simulink model "mod1"  (Simulink 8.9)
settings: Solver=ode45  StartTime=0.0  StopTime=simu.trantime  RelTol=1e-3  EnableMultiTasking=on
undefined symbols (not defined in the file): dc, Fs, mod, OSR, sinamp, sinfreq
libraries: dsparch4 x1, dspsrcs4 x1
settings Model: Creator=Isacco Arnaldi  LastModifiedBy=Arnaldi Isacco
settings SolverCC: AutoInsertRateTranBlk=on
settings DataIOCC: MaxDataPoints=50000  SaveOutput=off  SaveTime=off
settings OptimizationCC: DefaultParameterBehavior=Inlined  ExpressionDepthLimit=2147483647
settings DebuggingCC: SolverPrmCheckMsg=warning  StrictBusMsg=Warning

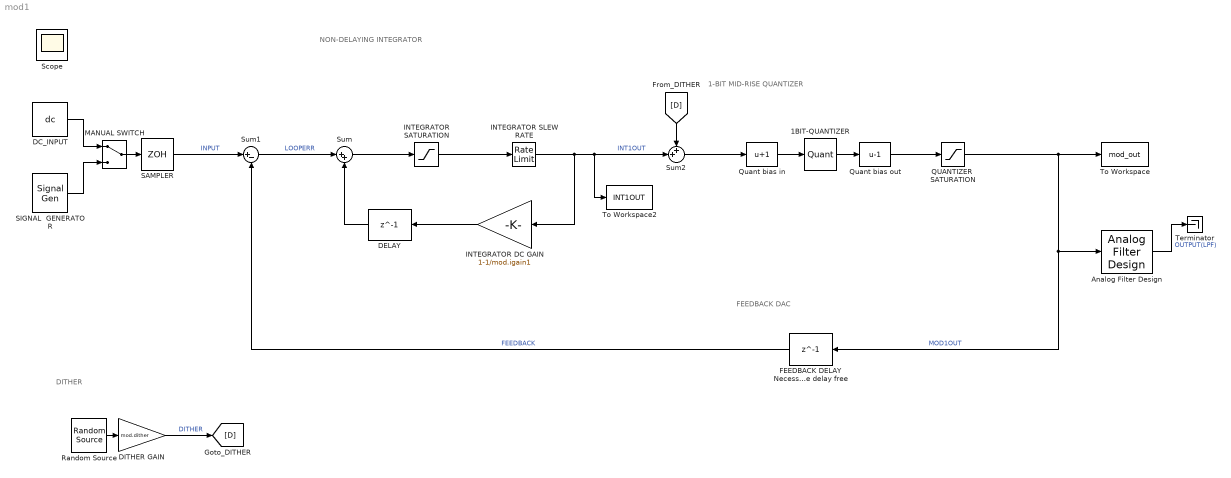
== system mod1 ==
  note: NON-DELAYING INTEGRATOR
  note: FEEDBACK DAC
  note: 1-BIT MID-RISE QUANTIZER
  note: DITHER
  1BIT-QUANTIZER : Quantizer  QuantizationInterval=2  LinearizeAsGain=off  SampleTime=1/Fs
      settings: AttributesFormatString=step = 2
  Analog Filter Design : dsparch4/Analog Filter Design  method=Butterworth  filttype=Lowpass  N=8  Wlo=pi*(Fs/OSR)  Whi=80  Rp=2  Rs=40
      settings: AttributesFormatString=Low-pass filter the loop output\nto illustrate intuitively how the\npulse density modulated +1/-1\noutput stream does indeed capture\nthe input signal
  DC_INPUT : Constant  Value=dc  OutDataTypeStr=double  SampleTime=1/Fs
  DELAY : Delay  DelayLength=1  InitialCondition=0  InputProcessing=Inherited
  DITHER GAIN : Gain  Gain=mod.dither  SampleTime=1/Fs
  FEEDBACK DELAY Necessary to avoid a delay-free loop as integrator and quantizer are delay free : Delay  DelayLength=1  InitialCondition=0  InputProcessing=Inherited
  INTEGRATOR SATURATION : Saturate  UpperLimit=mod.isat1  LowerLimit=-(mod.isat1)
      settings: AttributesFormatString=Real integrators will have\noutput swing limits (analog\nsignal headroom or digital\naccumulator min/max values)
  INTEGRATOR SLEW RATE : RateLimiter  RisingSlewLimit=mod.isr1  FallingSlewLimit=-(mod.isr1)  SampleTimeMode=inherited
      settings: AttributesFormatString=...and\nmay suffer from\npoor slew rate
  INTEGRATOR DC GAIN : Gain  Gain=1-1/mod.igain1
      settings: AttributesFormatString=Integrator leakage\n(model finite integrator dc/LF\ngain in analog modulators)
  MANUAL SWITCH : ManualSwitch
      settings: AttributesFormatString=Double click to\nselect the desired\ninput
  QUANTIZER  SATURATION : Saturate  UpperLimit=mod.qsatout1  LowerLimit=-(mod.qsatout1)
      settings: AttributesFormatString=Limit quantizer\noutput
  Quant bias in : Bias  Bias=1
      settings: AttributesFormatString=Need offset to give\nMID-RISE quantiser
  Quant bias out : Bias  Bias=-1
      settings: AttributesFormatString=Shift outputs to\n..., -2, 1, 1, ...
  Random Source : dspsrcs4/Random Source  SrcType=Uniform  NormMethod=Ziggurat  CltLength=12  MinVal=-1  MaxVal=1  MeanVal=0  VarVal=1  RepMode=Not repeatable  rawSeed=1  IsInherit=off  SampMode=Discrete  SampTime=1/Fs  SampFrame=1  DataType=Double  OutComplex=Real  OutputFrames=on
  SAMPLER : ZeroOrderHold  SampleTime=1/Fs
  SIGNAL  GENERATOR : SignalGenerator  Amplitude=sinamp  Frequency=sinfreq  VectorParams1D=off
  Sum : Sum  Inputs=|++
      settings: AttributesFormatString=Integrator\nsummer
  Sum1 : Sum  Inputs=|+-  SampleTime=1/Fs
      settings: AttributesFormatString=Modulator Input\nLoop Error (input - fbk)
  Sum2 : Sum  Inputs=++|
  Terminator : Terminator
  To Workspace : ToWorkspace  VariableName=mod_out  SampleTime=-1
      settings: AttributesFormatString=Export output to\nworkspace for\npost-processing
  To Workspace2 : ToWorkspace  VariableName=INT1OUT  SampleTime=-1
      settings: AttributesFormatString=Export output to\nworkspace for\npost-processing
  Scope : Scope
  wires:
  DELAY/1 -> Sum/2
  Sum/1 -> INTEGRATOR SATURATION/1
  Sum1/1 -> Sum/1  "LOOPERR"
  FEEDBACK DELAY Necessary to avoid a delay-free loop as integrator and quantizer are delay free/1 -> Sum1/2  "FEEDBACK"
  Random Source/1 -> DITHER GAIN/1
  INTEGRATOR DC GAIN/1 -> DELAY/1
  Quant bias out/1 -> QUANTIZER  SATURATION/1
  DITHER GAIN/1 -> [D]  "DITHER"
  Quant bias in/1 -> 1BIT-QUANTIZER/1
  1BIT-QUANTIZER/1 -> Quant bias out/1
  DC_INPUT/1 -> MANUAL SWITCH/1
  SIGNAL  GENERATOR/1 -> MANUAL SWITCH/2
  MANUAL SWITCH/1 -> SAMPLER/1
  Analog Filter Design/1 -> Terminator/1  "OUTPUT(LPF)"
  Sum2/1 -> Quant bias in/1
  [D] -> Sum2/1
  INTEGRATOR SLEW RATE/1 -> INTEGRATOR DC GAIN/1, To Workspace2/1, Sum2/2  "INT1OUT"
  INTEGRATOR SATURATION/1 -> INTEGRATOR SLEW RATE/1
  QUANTIZER  SATURATION/1 -> To Workspace/1, Analog Filter Design/1, FEEDBACK DELAY Necessary to avoid a delay-free loop as integrator and quantizer are delay free/1  "MOD1OUT"
  SAMPLER/1 -> Sum1/1  "INPUT"
